simulink model "DC_motor_speed"  (R2018a)
settings: Solver=VariableStepAuto  StartTime=0.0  StopTime=10.0  RelTol=1e-3
values from neighbouring files (symbols this model uses):
  b = 3.5077E-6    (= 3.5077e-06)    [DC_motor_position.m]    (also in DC_motor_speed_para.m = 0.1; cruise_control_para.m = 50)
  J = 3.2284E-6    (= 3.2284e-06)    [DC_motor_position.m]    (also in DC_motor_speed_para.m = 0.01)
  k = 0.01    [DC_motor_speed_para.m]    (also in Introduction_simulink_para.m = 1)
  L = 2.75E-6    (= 2.75e-06)    [DC_motor_position.m]    (also in DC_motor_speed_para.m = 0.5)
  R = 4    [DC_motor_position.m]    (also in DC_motor_speed_para.m = 1)
settings Model: Creator=Infi  LastModifiedBy=Infi

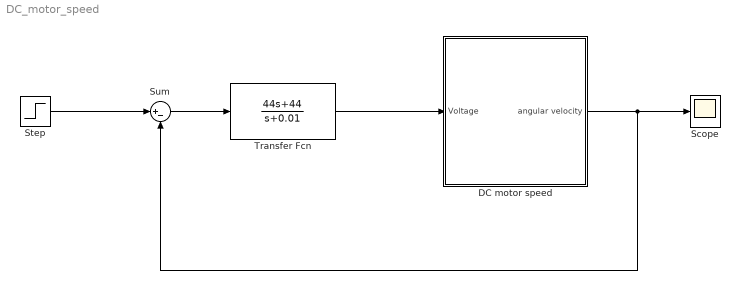
== system DC_motor_speed ==
  DC motor speed : Subsystem
  Scope : Scope
  Step : Step  SampleTime=0
  Sum : Sum  Inputs=|+-
  Transfer Fcn : TransferFcn  Numerator=[44 44]  Denominator=[1 0.01]
  wires:
  DC motor speed/1(angular velocity) -> Sum/2, Scope/1
  Transfer Fcn/1 -> DC motor speed/1(Voltage)
  Sum/1 -> Transfer Fcn/1
  Step/1 -> Sum/1

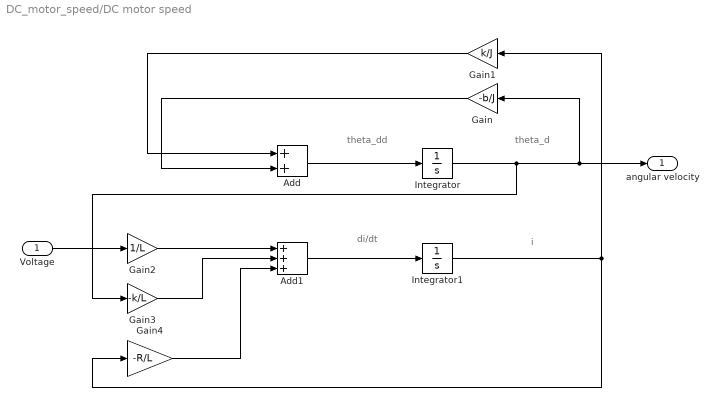
== system DC_motor_speed/DC motor speed ==
  note: theta_d
  note: i
  note: di/dt
  note: theta_dd
  Voltage : Inport
  Add : Sum
  Add1 : Sum  Inputs=+++
  Gain : Gain  Gain=-b/J
  Gain1 : Gain  Gain=k/J
  Gain2 : Gain  Gain=1/L
  Gain3 : Gain  Gain=-k/L
  Gain4 : Gain  Gain=-R/L
  Integrator : Integrator
  Integrator1 : Integrator
  angular velocity : Outport
  wires:
  Voltage/1 -> Gain2/1
  Gain1/1 -> Add/1
  Integrator/1 -> Gain3/1, angular velocity/1, Gain/1
  Gain/1 -> Add/2
  Gain4/1 -> Add1/3
  Gain3/1 -> Add1/2
  Integrator1/1 -> Gain4/1, Gain1/1
  Gain2/1 -> Add1/1
  Add/1 -> Integrator/1
  Add1/1 -> Integrator1/1
